simulink model "im_foc_1_1"  (R2022b)
settings: Solver=ode45  StartTime=0.0  StopTime=1  MaxStep=1e-4  MinStep=1e-5  RelTol=1e-4
values from neighbouring files (symbols this model uses):
  B = 0.00825    [IM_System_1.m]    (also in IM_System_2.m; IM_System_3.m; IM_System_noPU_4p2p2kw.m; IM_System_noPU_4p2p2kw_1.m)
  D = Ls*Lr - Lm^2    (= 0.000595276666667)    [IM_System_1.m]    (also in IM_System_2.m; IM_System_3.m; IM_System_noPU_4p2p2kw.m; IM_System_noPU_4p2p2kw_1.m)
  J = 0.013    [IM_System_1.m]    (also in IM_System_2.m; IM_System_3.m; IM_System_noPU_4p2p2kw.m; IM_System_noPU_4p2p2kw_1.m)
  Lm = 0.245/3    (= 0.0816666666667)    [IM_System_1.m]    (also in IM_System_2.m; IM_System_3.m; IM_System_noPU_4p2p2kw.m; IM_System_noPU_4p2p2kw_1.m)
  Lr = Ls    (= 0.0852333333333)    [IM_System_1.m]    (also in IM_System_2.m; IM_System_3.m; IM_System_noPU_4p2p2kw.m; IM_System_noPU_4p2p2kw_1.m)
  Ls = 0.2557/3    (= 0.0852333333333)    [IM_System_1.m]    (also in IM_System_2.m; IM_System_3.m; IM_System_noPU_4p2p2kw.m; IM_System_noPU_4p2p2kw_1.m)
  Lsigma = Ls - Lm^2/Lr    (= 0.00698408290966)    [IM_System_1.m]    (also in IM_System_2.m; IM_System_3.m; IM_System_noPU_4p2p2kw.m; IM_System_noPU_4p2p2kw_1.m)
  pole = 4    [im_params.m]
  Rr = 1.83/3    (= 0.61)    [IM_System_1.m]    (also in IM_System_2.m; IM_System_3.m; IM_System_noPU_4p2p2kw.m; IM_System_noPU_4p2p2kw_1.m)
  Rs = 2.5/3    (= 0.833333333333)    [IM_System_1.m]    (also in IM_System_2.m; IM_System_3.m; IM_System_noPU_4p2p2kw.m; IM_System_noPU_4p2p2kw_1.m)
  Tr = Lr/Rr    (= 0.139726775956)    [IM_System_1.m]    (also in IM_System_2.m; IM_System_3.m; IM_System_noPU_4p2p2kw.m; IM_System_noPU_4p2p2kw_1.m)
  w = w + iq_err*dt    (= -0.00016)    [IM_System_1.m]    (also in IM_System_2.m = -2e-05; IM_System_3.m = -2.2624e-05; IM_System_noPU_4p2p2kw.m = 0; IM_System_noPU_4p2p2kw_1.m = 0)
undefined symbols (not defined in the file or in its folder): DiscIntNeverNeededParam, sigbuilder_block, sigma
libraries: slpidlib x4
settings Model: Creator=jack  LastModifiedBy=jack

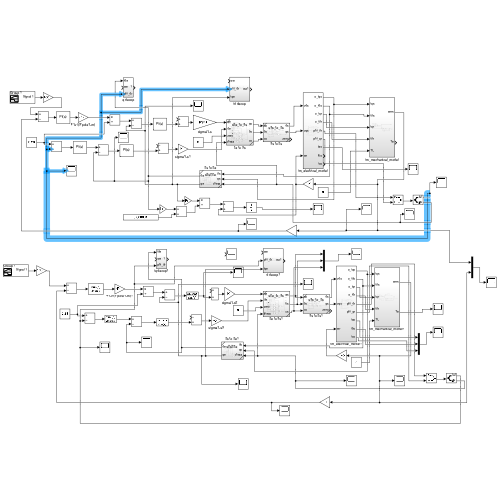
[thumbnail: Simulink's stored preview of the top-level diagram]
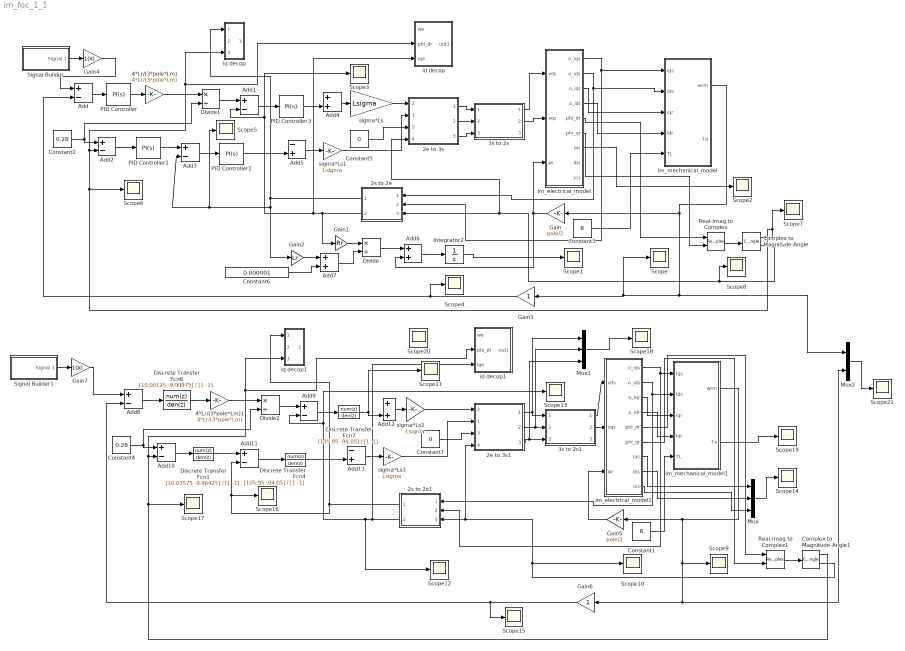
== system im_foc_1_1 ==
  2e to 3s : Subsystem  ReferencedSubsystem=s2e_to_3s
      settings: PortSchema="{\"entries\":[{\"content\":{\"sides\":[{\"content\":{\"connectorIds\":[\"In2\",\"In1\",\"In3\",\"In4\"]},\"type\":\"ConnectorPlacement.EquallySpacedRectSide\",\"uuid\":\"f133be33-91f9-49ed-9811-9ea3b8c2cc59\"},{\"content\":{\"connectorIds\":[\"Out1\",\"Out2\",\"Out3\"],\"side\":\"RIGHT\"},\"type\":\"ConnectorPlacement.EquallySpacedRectSide\",\"uuid\":\"fabe9076-6ecf-4b28-bd28-ced1febe4377\"},{\"content\":{\"connectorIds\":[],\"side\":\"TOP\"},\"type\":\"ConnectorPlacement.EquallySpacedRectSide\",\"uuid\":\"329e6c38-eee0-47c4-808c-a4969678c6ab\"}]},\"type\":\"ConnectorPlacement.EquallySpacedConnector\",\"uuid\":\"55c86aad-84a3-4804-b18d-62086c80b5dc\"}],\"packageUris\":[\"http://schema.mathworks.com/mf0/Connector/R2020b\"],\"version\":\"1.0\"}"
  2e to 3s1 : Subsystem  ReferencedSubsystem=s2e_to_3s
      settings: PortSchema="{\"entries\":[{\"content\":{\"sides\":[{\"content\":{\"connectorIds\":[\"In2\",\"In1\",\"In3\",\"In4\"]},\"type\":\"ConnectorPlacement.EquallySpacedRectSide\",\"uuid\":\"f133be33-91f9-49ed-9811-9ea3b8c2cc59\"},{\"content\":{\"connectorIds\":[\"Out1\",\"Out2\",\"Out3\"],\"side\":\"RIGHT\"},\"type\":\"ConnectorPlacement.EquallySpacedRectSide\",\"uuid\":\"fabe9076-6ecf-4b28-bd28-ced1febe4377\"},{\"content\":{\"connectorIds\":[],\"side\":\"TOP\"},\"type\":\"ConnectorPlacement.EquallySpacedRectSide\",\"uuid\":\"329e6c38-eee0-47c4-808c-a4969678c6ab\"}]},\"type\":\"ConnectorPlacement.EquallySpacedConnector\",\"uuid\":\"55c86aad-84a3-4804-b18d-62086c80b5dc\"}],\"packageUris\":[\"http://schema.mathworks.com/mf0/Connector/R2020b\"],\"version\":\"1.0\"}"
  2s to 2e : Subsystem  ReferencedSubsystem=s2s22e
  2s to 2e1 : Subsystem  ReferencedSubsystem=s2s22e
  3s to 2s : Subsystem  ReferencedSubsystem=s3s_to_2s
  3s to 2s1 : Subsystem  ReferencedSubsystem=s3s_to_2s
  4*Lr/(3*pole*Lm) : Gain  Gain=4*Lr/(3*pole*Lm)
  4*Lr/(3*pole*Lm)1 : Gain  Gain=4*Lr/(3*pole*Lm)
  Add{,1..3,8..11} (8 alike) : Sum  Inputs=+-
  Add{4,6..7,12} (4 alike) : Sum
  Add13 : Sum  Inputs=-+
  Add5 : Sum  Inputs=-+
  Complex to Magnitude-Angle : ComplexToMagnitudeAngle
  Complex to Magnitude-Angle1 : ComplexToMagnitudeAngle
  Constant1 : Constant  Value=8
  Constant2 : Constant  Value=0.28
  Constant3 : Constant  Value=8
  Constant4 : Constant  Value=0.28
  Constant5 : Constant  Value=0
  Constant6 : Constant  Value=0.000001
  Constant7 : Constant  Value=0
  Discrete Transfer Fcn1 : DiscreteTransferFcn  Numerator=[10.03575 -9.96425]  Denominator=[1 -1]  SampleTime=0.001
  Discrete Transfer Fcn4 : DiscreteTransferFcn  Numerator=[105.95 -94.05]  Denominator=[1 -1]  SampleTime=0.001
  Discrete Transfer Fcn7 : DiscreteTransferFcn  Numerator=[105.95 -94.05]  Denominator=[1 -1]  SampleTime=0.001
  Discrete Transfer Fcn8 : DiscreteTransferFcn  Numerator=[10.00125 -9.99875]  Denominator=[1 -1]  SampleTime=0.001
  Divide : Product  Inputs=*/
  Divide1 : Product  Inputs=*/
  Divide2 : Product  Inputs=*/
  Gain : Gain  Gain=pole/2
  Gain1 : Gain  Gain=Rr
  Gain2 : Gain  Gain=Lr
  Gain3 : Gain
  Gain4 : Gain  Gain=100
  Gain5 : Gain  Gain=pole/2
  Gain6 : Gain
  Gain7 : Gain  Gain=100
  Integrator2 : Integrator
  Mux : Mux  Inputs=3
  Mux1 : Mux  Inputs=3
  Mux2 : Mux  Inputs=2
  PID Controller : slpidlib/PID Controller  Controller=PI  Form=Parallel  TimeDomain=Continuous-time  UseExternalTs=off  SampleTime=-1  IntegratorMethod=Forward Euler  FilterMethod=Forward Euler  ControllerParametersSource=internal  P=10  I=0.25*10  UseKiTs=off  D=0  N=100  UseFilter=on  TunerSelectOption=Transfer Function Based (PID Tuner App)  InitialConditionSource=internal  InitialConditionForIntegrator=0  InitialConditionForFilter=0  DifferentiatorICPrevScaledInput=0  ExternalReset=none  TrackingMode=off  Kt=1  LimitOutput=off  SatLimitsSource=internal  UpperSaturationLimit=inf  LowerSaturationLimit=-inf  LinearizeAsGain=on  AntiWindupMode=none  Kb=1  LimitIntegrator=off  UpperIntegratorSaturationLimit=inf  LowerIntegratorSaturationLimit=-inf  POutMin=[]  POutMax=[]  IOutMin=[]  IOutMax=[]  DOutMin=[]  DOutMax=[]  NOutMin=[]  NOutMax=[]  SumOutMin=[]  SumOutMax=[]  SaturationOutMin=[]  SaturationOutMax=[]  PParamMin=[]  PParamMax=[]  IParamMin=[]  IParamMax=[]  DParamMin=[]  DParamMax=[]  NParamMin=[]  NParamMax=[]  KbParamMin=[]  KbParamMax=[]  KtParamMin=[]  KtParamMax=[]  KbOutMin=[]  KbOutMax=[]  KtOutMin=[]  KtOutMax=[]  IntegratorOutMin=[]  IntegratorOutMax=[]  FilterOutMin=[]  FilterOutMax=[]  SumI1OutMin=[]  SumI1OutMax=[]  SumI2OutMin=[]  SumI2OutMax=[]  SumI3OutMin=[]  SumI3OutMax=[]  SumI4OutMin=[]  SumI4OutMax=[]  SumDOutMin=[]  SumDOutMax=[]  DifferentiatorOutMin=[]  DifferentiatorOutMax=[]  FilterDiffOutCoefMin=[]  FilterDiffOutCoefMax=[]  ReciprocalOutMin=[]  ReciprocalOutMax=[]  SumDenOutMin=[]  SumDenOutMax=[]  SumNumOutMin=[]  SumNumOutMax=[]  DivideOutMin=[]  DivideOutMax=[]  UdiffTsProdOutMin=[]  UdiffTsProdOutMax=[]  NTsProdOutMin=[]  NTsProdOutMax=[]  UintegralTsProdOutMin=[]  UintegralTsProdOutMax=[]  UngainTsProdOutMin=[]  UngainTsProdOutMax=[]  ClampingZeroOutDataTypeStr=Inherit: Inherit via back propagation  ClampingZeroOutMin=[]  ClampingZeroOutMax=[]  FilterDenConstantOutDataTypeStr=Inherit: Inherit via back propagation  FilterDenConstantOutMin=[]  FilterDenConstantOutMax=[]  PCopyOutDataTypeStr=Inherit: Inherit via back propagation  PCopyOutMin=[]  PCopyOutMax=[]  NCopyOutDataTypeStr=Inherit: Inherit via back propagation  NCopyOutMin=[]  NCopyOutMax=[]  IntegratorContinuousStateAttributes=''  IntegratorStateMustResolveToSignalObject=off  IntegratorRTWStateStorageClass=Auto  FilterContinuousStateAttributes=''  FilterStateMustResolveToSignalObject=off  FilterRTWStateStorageClass=Auto  ParallelPVariant=InternalParameters  IdealPVariant=Disabled  IVariant=InternalParameters  DVariant=Disabled  IntegratorVariant=Continuous  SatVariant=Disabled  AWVariant=Passthrough  PCopyVariant=Disabled  TRVariant=Disabled  FdbkBlocksVariant=Forward  IdealPFdbkVariant=Disabled  SatFdbkVariant=Disabled  DerivativeFilterVariant=Disabled  NVariant=Disabled  NCopyVariant=Disabled_SignalSpec  FilterICVariant=Disabled  IntegratorICVariant=InternalICs  ExternalResetVariant=Disabled  TRSumVariant=Passthrough  SumFdbkVariant=Disabled  SumVariant=Sum_PI  TsampFilterVariant=InternalTs  TsampNgainVariant=Passthrough  TsampIntegralVariant=Passthrough  ExternalSaturationOutDataTypeStr=Inherit: Same as second input
  PID Controller1 : slpidlib/PID Controller  Controller=PI  Form=Parallel  TimeDomain=Continuous-time  UseExternalTs=off  SampleTime=-1  IntegratorMethod=Forward Euler  FilterMethod=Forward Euler  ControllerParametersSource=internal  P=10  I=7.15*10  UseKiTs=off  D=0  N=100  UseFilter=on  TunerSelectOption=Transfer Function Based (PID Tuner App)  InitialConditionSource=internal  InitialConditionForIntegrator=0  InitialConditionForFilter=0  DifferentiatorICPrevScaledInput=0  ExternalReset=none  TrackingMode=off  Kt=1  LimitOutput=off  SatLimitsSource=internal  UpperSaturationLimit=inf  LowerSaturationLimit=-inf  LinearizeAsGain=on  AntiWindupMode=none  Kb=1  LimitIntegrator=off  UpperIntegratorSaturationLimit=inf  LowerIntegratorSaturationLimit=-inf  POutMin=[]  POutMax=[]  IOutMin=[]  IOutMax=[]  DOutMin=[]  DOutMax=[]  NOutMin=[]  NOutMax=[]  SumOutMin=[]  SumOutMax=[]  SaturationOutMin=[]  SaturationOutMax=[]  PParamMin=[]  PParamMax=[]  IParamMin=[]  IParamMax=[]  DParamMin=[]  DParamMax=[]  NParamMin=[]  NParamMax=[]  KbParamMin=[]  KbParamMax=[]  KtParamMin=[]  KtParamMax=[]  KbOutMin=[]  KbOutMax=[]  KtOutMin=[]  KtOutMax=[]  IntegratorOutMin=[]  IntegratorOutMax=[]  FilterOutMin=[]  FilterOutMax=[]  SumI1OutMin=[]  SumI1OutMax=[]  SumI2OutMin=[]  SumI2OutMax=[]  SumI3OutMin=[]  SumI3OutMax=[]  SumI4OutMin=[]  SumI4OutMax=[]  SumDOutMin=[]  SumDOutMax=[]  DifferentiatorOutMin=[]  DifferentiatorOutMax=[]  FilterDiffOutCoefMin=[]  FilterDiffOutCoefMax=[]  ReciprocalOutMin=[]  ReciprocalOutMax=[]  SumDenOutMin=[]  SumDenOutMax=[]  SumNumOutMin=[]  SumNumOutMax=[]  DivideOutMin=[]  DivideOutMax=[]  UdiffTsProdOutMin=[]  UdiffTsProdOutMax=[]  NTsProdOutMin=[]  NTsProdOutMax=[]  UintegralTsProdOutMin=[]  UintegralTsProdOutMax=[]  UngainTsProdOutMin=[]  UngainTsProdOutMax=[]  ClampingZeroOutDataTypeStr=Inherit: Inherit via back propagation  ClampingZeroOutMin=[]  ClampingZeroOutMax=[]  FilterDenConstantOutDataTypeStr=Inherit: Inherit via back propagation  FilterDenConstantOutMin=[]  FilterDenConstantOutMax=[]  PCopyOutDataTypeStr=Inherit: Inherit via back propagation  PCopyOutMin=[]  PCopyOutMax=[]  NCopyOutDataTypeStr=Inherit: Inherit via back propagation  NCopyOutMin=[]  NCopyOutMax=[]  IntegratorContinuousStateAttributes=''  IntegratorStateMustResolveToSignalObject=off  IntegratorRTWStateStorageClass=Auto  FilterContinuousStateAttributes=''  FilterStateMustResolveToSignalObject=off  FilterRTWStateStorageClass=Auto  ParallelPVariant=InternalParameters  IdealPVariant=Disabled  IVariant=InternalParameters  DVariant=Disabled  IntegratorVariant=Continuous  SatVariant=Disabled  AWVariant=Passthrough  PCopyVariant=Disabled  TRVariant=Disabled  FdbkBlocksVariant=Forward  IdealPFdbkVariant=Disabled  SatFdbkVariant=Disabled  DerivativeFilterVariant=Disabled  NVariant=Disabled  NCopyVariant=Disabled_SignalSpec  FilterICVariant=Disabled  IntegratorICVariant=InternalICs  ExternalResetVariant=Disabled  TRSumVariant=Passthrough  SumFdbkVariant=Disabled  SumVariant=Sum_PI  TsampFilterVariant=InternalTs  TsampNgainVariant=Passthrough  TsampIntegralVariant=Passthrough  ExternalSaturationOutDataTypeStr=Inherit: Same as second input
  PID Controller2 : slpidlib/PID Controller  Controller=PI  Form=Parallel  TimeDomain=Continuous-time  UseExternalTs=off  SampleTime=-1  IntegratorMethod=Forward Euler  FilterMethod=Forward Euler  ControllerParametersSource=internal  P=100  I=119*100  UseKiTs=off  D=0  N=100  UseFilter=on  TunerSelectOption=Transfer Function Based (PID Tuner App)  InitialConditionSource=internal  InitialConditionForIntegrator=0  InitialConditionForFilter=0  DifferentiatorICPrevScaledInput=0  ExternalReset=none  TrackingMode=off  Kt=1  LimitOutput=off  SatLimitsSource=internal  UpperSaturationLimit=inf  LowerSaturationLimit=-inf  LinearizeAsGain=on  AntiWindupMode=none  Kb=1  LimitIntegrator=off  UpperIntegratorSaturationLimit=inf  LowerIntegratorSaturationLimit=-inf  POutMin=[]  POutMax=[]  IOutMin=[]  IOutMax=[]  DOutMin=[]  DOutMax=[]  NOutMin=[]  NOutMax=[]  SumOutMin=[]  SumOutMax=[]  SaturationOutMin=[]  SaturationOutMax=[]  PParamMin=[]  PParamMax=[]  IParamMin=[]  IParamMax=[]  DParamMin=[]  DParamMax=[]  NParamMin=[]  NParamMax=[]  KbParamMin=[]  KbParamMax=[]  KtParamMin=[]  KtParamMax=[]  KbOutMin=[]  KbOutMax=[]  KtOutMin=[]  KtOutMax=[]  IntegratorOutMin=[]  IntegratorOutMax=[]  FilterOutMin=[]  FilterOutMax=[]  SumI1OutMin=[]  SumI1OutMax=[]  SumI2OutMin=[]  SumI2OutMax=[]  SumI3OutMin=[]  SumI3OutMax=[]  SumI4OutMin=[]  SumI4OutMax=[]  SumDOutMin=[]  SumDOutMax=[]  DifferentiatorOutMin=[]  DifferentiatorOutMax=[]  FilterDiffOutCoefMin=[]  FilterDiffOutCoefMax=[]  ReciprocalOutMin=[]  ReciprocalOutMax=[]  SumDenOutMin=[]  SumDenOutMax=[]  SumNumOutMin=[]  SumNumOutMax=[]  DivideOutMin=[]  DivideOutMax=[]  UdiffTsProdOutMin=[]  UdiffTsProdOutMax=[]  NTsProdOutMin=[]  NTsProdOutMax=[]  UintegralTsProdOutMin=[]  UintegralTsProdOutMax=[]  UngainTsProdOutMin=[]  UngainTsProdOutMax=[]  ClampingZeroOutDataTypeStr=Inherit: Inherit via back propagation  ClampingZeroOutMin=[]  ClampingZeroOutMax=[]  FilterDenConstantOutDataTypeStr=Inherit: Inherit via back propagation  FilterDenConstantOutMin=[]  FilterDenConstantOutMax=[]  PCopyOutDataTypeStr=Inherit: Inherit via back propagation  PCopyOutMin=[]  PCopyOutMax=[]  NCopyOutDataTypeStr=Inherit: Inherit via back propagation  NCopyOutMin=[]  NCopyOutMax=[]  IntegratorContinuousStateAttributes=''  IntegratorStateMustResolveToSignalObject=off  IntegratorRTWStateStorageClass=Auto  FilterContinuousStateAttributes=''  FilterStateMustResolveToSignalObject=off  FilterRTWStateStorageClass=Auto  ParallelPVariant=InternalParameters  IdealPVariant=Disabled  IVariant=InternalParameters  DVariant=Disabled  IntegratorVariant=Continuous  SatVariant=Disabled  AWVariant=Passthrough  PCopyVariant=Disabled  TRVariant=Disabled  FdbkBlocksVariant=Forward  IdealPFdbkVariant=Disabled  SatFdbkVariant=Disabled  DerivativeFilterVariant=Disabled  NVariant=Disabled  NCopyVariant=Disabled_SignalSpec  FilterICVariant=Disabled  IntegratorICVariant=InternalICs  ExternalResetVariant=Disabled  TRSumVariant=Passthrough  SumFdbkVariant=Disabled  SumVariant=Sum_PI  TsampFilterVariant=InternalTs  TsampNgainVariant=Passthrough  TsampIntegralVariant=Passthrough  ExternalSaturationOutDataTypeStr=Inherit: Same as second input
  PID Controller3 : slpidlib/PID Controller  Controller=PI  Form=Parallel  TimeDomain=Continuous-time  UseExternalTs=off  SampleTime=-1  IntegratorMethod=Forward Euler  FilterMethod=Forward Euler  ControllerParametersSource=internal  P=100  I=119*100  UseKiTs=off  D=0  N=100  UseFilter=on  TunerSelectOption=Transfer Function Based (PID Tuner App)  InitialConditionSource=internal  InitialConditionForIntegrator=0  InitialConditionForFilter=0  DifferentiatorICPrevScaledInput=0  ExternalReset=none  TrackingMode=off  Kt=1  LimitOutput=off  SatLimitsSource=internal  UpperSaturationLimit=inf  LowerSaturationLimit=-inf  LinearizeAsGain=on  AntiWindupMode=none  Kb=1  LimitIntegrator=off  UpperIntegratorSaturationLimit=inf  LowerIntegratorSaturationLimit=-inf  POutMin=[]  POutMax=[]  IOutMin=[]  IOutMax=[]  DOutMin=[]  DOutMax=[]  NOutMin=[]  NOutMax=[]  SumOutMin=[]  SumOutMax=[]  SaturationOutMin=[]  SaturationOutMax=[]  PParamMin=[]  PParamMax=[]  IParamMin=[]  IParamMax=[]  DParamMin=[]  DParamMax=[]  NParamMin=[]  NParamMax=[]  KbParamMin=[]  KbParamMax=[]  KtParamMin=[]  KtParamMax=[]  KbOutMin=[]  KbOutMax=[]  KtOutMin=[]  KtOutMax=[]  IntegratorOutMin=[]  IntegratorOutMax=[]  FilterOutMin=[]  FilterOutMax=[]  SumI1OutMin=[]  SumI1OutMax=[]  SumI2OutMin=[]  SumI2OutMax=[]  SumI3OutMin=[]  SumI3OutMax=[]  SumI4OutMin=[]  SumI4OutMax=[]  SumDOutMin=[]  SumDOutMax=[]  DifferentiatorOutMin=[]  DifferentiatorOutMax=[]  FilterDiffOutCoefMin=[]  FilterDiffOutCoefMax=[]  ReciprocalOutMin=[]  ReciprocalOutMax=[]  SumDenOutMin=[]  SumDenOutMax=[]  SumNumOutMin=[]  SumNumOutMax=[]  DivideOutMin=[]  DivideOutMax=[]  UdiffTsProdOutMin=[]  UdiffTsProdOutMax=[]  NTsProdOutMin=[]  NTsProdOutMax=[]  UintegralTsProdOutMin=[]  UintegralTsProdOutMax=[]  UngainTsProdOutMin=[]  UngainTsProdOutMax=[]  ClampingZeroOutDataTypeStr=Inherit: Inherit via back propagation  ClampingZeroOutMin=[]  ClampingZeroOutMax=[]  FilterDenConstantOutDataTypeStr=Inherit: Inherit via back propagation  FilterDenConstantOutMin=[]  FilterDenConstantOutMax=[]  PCopyOutDataTypeStr=Inherit: Inherit via back propagation  PCopyOutMin=[]  PCopyOutMax=[]  NCopyOutDataTypeStr=Inherit: Inherit via back propagation  NCopyOutMin=[]  NCopyOutMax=[]  IntegratorContinuousStateAttributes=''  IntegratorStateMustResolveToSignalObject=off  IntegratorRTWStateStorageClass=Auto  FilterContinuousStateAttributes=''  FilterStateMustResolveToSignalObject=off  FilterRTWStateStorageClass=Auto  ParallelPVariant=InternalParameters  IdealPVariant=Disabled  IVariant=InternalParameters  DVariant=Disabled  IntegratorVariant=Continuous  SatVariant=Disabled  AWVariant=Passthrough  PCopyVariant=Disabled  TRVariant=Disabled  FdbkBlocksVariant=Forward  IdealPFdbkVariant=Disabled  SatFdbkVariant=Disabled  DerivativeFilterVariant=Disabled  NVariant=Disabled  NCopyVariant=Disabled_SignalSpec  FilterICVariant=Disabled  IntegratorICVariant=InternalICs  ExternalResetVariant=Disabled  TRSumVariant=Passthrough  SumFdbkVariant=Disabled  SumVariant=Sum_PI  TsampFilterVariant=InternalTs  TsampNgainVariant=Passthrough  TsampIntegralVariant=Passthrough  ExternalSaturationOutDataTypeStr=Inherit: Same as second input
  Real-Imag to Complex : RealImagToComplex
  Real-Imag to Complex1 : RealImagToComplex
  Scope{,1..21} (22 alike) : Scope
  Signal Builder : Subsystem  Tag=STV Subsys  LoadFcn=sigbuilder_block('load');  StartFcn=sigbuilder_block('start');  StopFcn=sigbuilder_block('stop');  ClipboardFcn=sigbuilder_block('clipboard');  mask(Sigbuilder block){tuvar=[0:10]}
      mask help: Simulink:masks:SigbuilderBlock_MD
      mask init:
      | if ~strcmp(get_param(bdroot(gcbh),'SimulationStatus'),'stopped') tuvar = sigbuilder_block('maskInit'); end
      settings: CopyFcn=sigbuilder_block('copy');  DeleteFcn=sigbuilder_block('delete');  ModelCloseFcn=sigbuilder_block('modelClose');  PreSaveFcn=sigbuilder_block('preSave');  PauseFcn=sigbuilder_block('pause');  ContinueFcn=sigbuilder_block('continue');  NameChangeFcn=sigbuilder_block('namechange');  OpenFcn=sigbuilder_block('open',[437.6 199.2 550.4 400 ]);  CloseFcn=sigbuilder_block('close');
      mask Display: plot(0, 0, 100, 100,[2, 2, 32, 32, 2], [68, 8, 8, 68, 68],[32, 2], [38, 38], [32, 19, 2],[53, 60, 44], [32, 17, 17, 2],[16, 16, 31, 31]);txt = getActiveGroup(gcbh);text(2, 100, txt,'verticalAlignment', 'top');
  Signal Builder1 : Subsystem  Tag=STV Subsys  LoadFcn=sigbuilder_block('load');  StartFcn=sigbuilder_block('start');  StopFcn=sigbuilder_block('stop');  ClipboardFcn=sigbuilder_block('clipboard');  mask(Sigbuilder block){tuvar=[0:10]}
      mask help: Simulink:masks:SigbuilderBlock_MD
      mask init:
      | if ~strcmp(get_param(bdroot(gcbh),'SimulationStatus'),'stopped') tuvar = sigbuilder_block('maskInit'); end
      settings: CopyFcn=sigbuilder_block('copy');  DeleteFcn=sigbuilder_block('delete');  ModelCloseFcn=sigbuilder_block('modelClose');  PreSaveFcn=sigbuilder_block('preSave');  PauseFcn=sigbuilder_block('pause');  ContinueFcn=sigbuilder_block('continue');  NameChangeFcn=sigbuilder_block('namechange');  OpenFcn=sigbuilder_block('open',[437.6 199.2 550.4 400 ]);  CloseFcn=sigbuilder_block('close');
      mask Display: plot(0, 0, 100, 100,[2, 2, 32, 32, 2], [68, 8, 8, 68, 68],[32, 2], [38, 38], [32, 19, 2],[53, 60, 44], [32, 17, 17, 2],[16, 16, 31, 31]);txt = getActiveGroup(gcbh);text(2, 100, txt,'verticalAlignment', 'top');
  id decop : Subsystem
  id decop1 : Subsystem
  im_electrical_model : Subsystem
  im_electrical_model1 : Subsystem
  im_mechanical_model : Subsystem
  im_mechanical_model1 : Subsystem
  iq decop : Subsystem
  iq decop1 : Subsystem
  sigma*Ls{,1..3} (4 alike) : Gain  Gain=Lsigma
  wires:
  Add/1 -> PID Controller/1
  4*Lr/(3*pole*Lm)/1 -> Divide1/1
  PID Controller/1 -> 4*Lr/(3*pole*Lm)/1
  Divide1/1 -> Add1/1
  Constant2/1 -> Add2/1, Divide1/2
  Add2/1 -> PID Controller1/1
  PID Controller1/1 -> Add3/1
  Add3/1 -> PID Controller2/1
  Add1/1 -> PID Controller3/1
  PID Controller3/1 -> Add4/2
  Add4/1 -> sigma*Ls/1
  sigma*Ls/1 -> 2e to 3s/2
  PID Controller2/1 -> Add5/2
  Add5/1 -> sigma*Ls1/1
  sigma*Ls1/1 -> 2e to 3s/1
  3s to 2s/1 -> im_electrical_model/1(vds)
  3s to 2s/2 -> im_electrical_model/2(vqs)
  im_mechanical_model/1(wrm) -> Gain/1, Scope/1, Gain3/1, Mux2/1
  im_electrical_model/1(o_iqs) -> im_mechanical_model/1(iqs), 2s to 2e/2
  im_electrical_model/2(o_ids) -> 2s to 2e/1, im_mechanical_model/2(ids)
  im_electrical_model/3(o_iqr) -> im_mechanical_model/3(iqr)
  im_electrical_model/4(o_idr) -> im_mechanical_model/4(idr)
  2s to 2e/1 -> iq decop/1(ide), Gain2/1, Scope5/1, Add3/2
  2s to 2e/2 -> id decop/3(iqe), Scope3/1, Add1/2, Gain1/1
  Gain1/1 -> Divide/1
  Divide/1 -> Add6/1
  Gain/1 -> im_electrical_model/3(wr), Add6/2
  Add6/1 -> Integrator2/1
  Integrator2/1 -> Scope1/1
  Constant5/1 -> 2e to 3s/3
  Gain2/1 -> Add7/1
  Add7/1 -> Divide/2
  Constant6/1 -> Add7/2
  2e to 3s/1 -> 3s to 2s/1
  2e to 3s/3 -> 3s to 2s/3
  im_electrical_model/7(ias) -> Scope2/1
  Gain3/1 -> Scope4/1, Add/2
  2e to 3s/2 -> 3s to 2s/2
  Signal Builder/1(Signal 1) -> Gain4/1
  Complex to Magnitude-Angle/1 -> Scope6/1, id decop/2(phi_dr), iq decop/3(phi_dr), Add2/2, Scope7/1
  Constant3/1 -> im_mechanical_model/5(TL)
  Gain4/1 -> Add/1
  im_electrical_model/5(phi_dr) -> Real-Imag to Complex/1
  im_electrical_model/6(phi_qr) -> Real-Imag to Complex/2
  Real-Imag to Complex/1 -> Complex to Magnitude-Angle/1
  Complex to Magnitude-Angle/2 -> Scope8/1, 2e to 3s/4, 2s to 2e/3
  Real-Imag to Complex1/1 -> Complex to Magnitude-Angle1/1
  3s to 2s1/2 -> im_electrical_model1/2(vqs)
  Signal Builder1/1(Signal 1) -> Gain7/1
  Constant4/1 -> Add10/1, Divide2/2
  im_electrical_model1/3(o_iqr) -> im_mechanical_model1/3(iqr)
  Discrete Transfer Fcn1/1 -> Add11/1
  im_electrical_model1/1(o_iqs) -> im_mechanical_model1/1(iqs), 2s to 2e1/2
  im_electrical_model1/5(phi_dr) -> Real-Imag to Complex1/1
  2s to 2e1/2 -> Scope12/1, Scope13/1, Add9/2, id decop1/3(iqe)
  Add9/1 -> Discrete Transfer Fcn7/1
  im_mechanical_model1/1(wrm) -> Gain5/1, Gain6/1, Mux2/2, Scope9/1
  2s to 2e1/1 -> iq decop1/1(ide), Scope16/1, Add11/2
  im_electrical_model1/2(o_ids) -> 2s to 2e1/1, im_mechanical_model1/2(ids)
  Discrete Transfer Fcn4/1 -> Add13/2
  Add12/1 -> sigma*Ls2/1
  2e to 3s1/1 -> Mux1/1, 3s to 2s1/1
  Add8/1 -> Discrete Transfer Fcn8/1
  4*Lr/(3*pole*Lm)1/1 -> Divide2/1
  Constant1/1 -> im_mechanical_model1/5(TL)
  Add13/1 -> sigma*Ls3/1
  im_electrical_model1/4(o_idr) -> im_mechanical_model1/4(idr)
  Discrete Transfer Fcn7/1 -> Scope11/1, Add12/2
  Gain5/1 -> im_electrical_model1/3(wr)
  sigma*Ls2/1 -> 2e to 3s1/2
  Constant7/1 -> 2e to 3s1/3
  Add10/1 -> Discrete Transfer Fcn1/1
  Complex to Magnitude-Angle1/2 -> 2e to 3s1/4, 2s to 2e1/3, Scope10/1
  im_electrical_model1/9(ics) -> Mux/3
  Add11/1 -> Discrete Transfer Fcn4/1
  2e to 3s1/3 -> Mux1/3, 3s to 2s1/3
  im_electrical_model1/7(ias) -> Mux/1
  im_electrical_model1/6(phi_qr) -> Real-Imag to Complex1/2
  im_electrical_model1/8(ibs) -> Mux/2
  Mux/1 -> Scope14/1
  Discrete Transfer Fcn8/1 -> 4*Lr/(3*pole*Lm)1/1
  Mux1/1 -> Scope18/1
  Gain6/1 -> Scope15/1, Add8/2
  3s to 2s1/1 -> im_electrical_model1/1(vds)
  Gain7/1 -> Add8/1
  2e to 3s1/2 -> Mux1/2, 3s to 2s1/2
  im_mechanical_model1/2(Te) -> Scope19/1
  Divide2/1 -> Add9/1
  Complex to Magnitude-Angle1/1 -> Scope17/1, id decop1/2(phi_dr), iq decop1/3(phi_dr), Add10/2
  sigma*Ls3/1 -> 2e to 3s1/1
  Mux2/1 -> Scope21/1

== system im_foc_1_1/Signal Builder ==
  Demux : Demux  Tag=STV Demux  Outputs=1
      settings: DisplayOption=none
  FromWs : FromWorkspace  Tag=STV FromWs  VariableName=tuvar
      SigBuilderData=|
      | common.afterFinalStr = 'Extrapolate'
      | common.sampleTime = 0
      | dataSet.timeRange = [0 10]
      | dataSet.name = 'Group 1'
      | sbobj.Groups.Name = 'Group 1'
      | sbobj.Groups.Signals.Name = 'Signal 1'
      | sbobj.Groups.Signals.XData = [0 0.5 4 6 6 10]
      | sbobj.Groups.Signals.YData = [0 1 1 1 0 0]
  Signal 1 : Outport  Tag=STV Outport
  wires:
  Demux/1 -> Signal 1/1
  FromWs/1 -> Demux/1

== system im_foc_1_1/Signal Builder1 ==
  Demux : Demux  Tag=STV Demux  Outputs=1
      settings: DisplayOption=none
  FromWs : FromWorkspace  Tag=STV FromWs  VariableName=tuvar
      SigBuilderData=|
      | common.afterFinalStr = 'Extrapolate'
      | common.sampleTime = 0
      | dataSet.timeRange = [0 10]
      | dataSet.name = 'Group 1'
      | sbobj.Groups.Name = 'Group 1'
      | sbobj.Groups.Signals.Name = 'Signal 1'
      | sbobj.Groups.Signals.XData = [0 0.5 4 6 6 10]
      | sbobj.Groups.Signals.YData = [0 1 1 1 0 0]
  Signal 1 : Outport  Tag=STV Outport
  wires:
  Demux/1 -> Signal 1/1
  FromWs/1 -> Demux/1

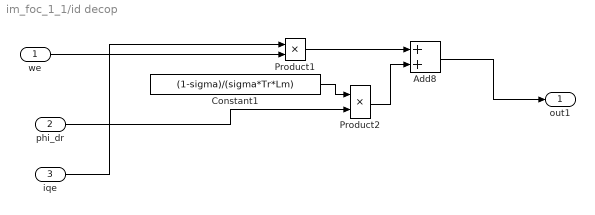
== system im_foc_1_1/id decop ==
  we : Inport
  phi_dr : Inport  Port=2
  iqe : Inport  Port=3
  Add8 : Sum
  Constant1 : Constant  Value=(1-sigma)/(sigma*Tr*Lm)
  Product1 : Product
  Product2 : Product
  out1 : Outport
  wires:
  Product1/1 -> Add8/1
  iqe/1 -> Product1/1
  Add8/1 -> out1/1
  we/1 -> Product1/2
  Constant1/1 -> Product2/1
  Product2/1 -> Add8/2
  phi_dr/1 -> Product2/2

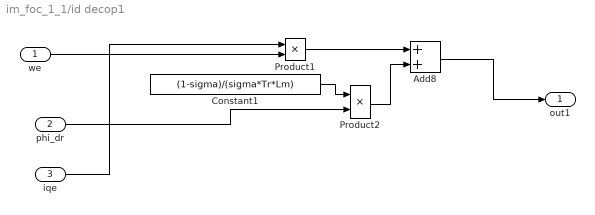
== system im_foc_1_1/id decop1 ==
  we : Inport
  phi_dr : Inport  Port=2
  iqe : Inport  Port=3
  Add8 : Sum
  Constant1 : Constant  Value=(1-sigma)/(sigma*Tr*Lm)
  Product1 : Product
  Product2 : Product
  out1 : Outport
  wires:
  Product1/1 -> Add8/1
  iqe/1 -> Product1/1
  Add8/1 -> out1/1
  we/1 -> Product1/2
  Constant1/1 -> Product2/1
  Product2/1 -> Add8/2
  phi_dr/1 -> Product2/2

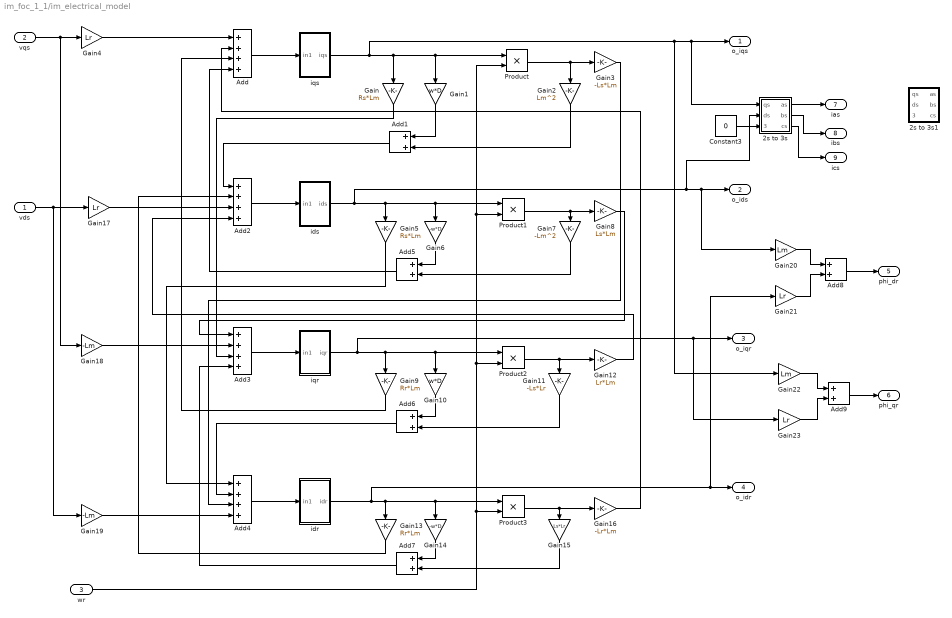
== system im_foc_1_1/im_electrical_model ==
  vds : Inport
  vqs : Inport  Port=2
  wr : Inport  Port=3
  2s to 3s : Subsystem
  2s to 3s1 : Subsystem
  Add{,2..4} (4 alike) : Sum  Inputs=++++
  Add{1,5..9} (6 alike) : Sum
  Constant3 : Constant  Value=0
  Gain : Gain  Gain=Rs*Lm
  Gain1 : Gain  Gain=w*D
  Gain10 : Gain  Gain=w*D
  Gain11 : Gain  Gain=-Ls*Lr
  Gain12 : Gain  Gain=Lr*Lm
  Gain13 : Gain  Gain=Rr*Lm
  Gain14 : Gain  Gain=-w*D
  Gain15 : Gain  Gain=Ls*Lr
  Gain16 : Gain  Gain=-Lr*Lm
  Gain{4,17,21,23} (4 alike) : Gain  Gain=Lr
  Gain18 : Gain  Gain=-Lm
  Gain19 : Gain  Gain=-Lm
  Gain2 : Gain  Gain=Lm^2
  Gain20 : Gain  Gain=Lm
  Gain22 : Gain  Gain=Lm
  Gain3 : Gain  Gain=-Ls*Lm
  Gain5 : Gain  Gain=Rs*Lm
  Gain6 : Gain  Gain=-w*D
  Gain7 : Gain  Gain=-Lm^2
  Gain8 : Gain  Gain=Ls*Lm
  Gain9 : Gain  Gain=Rr*Lm
  Product{,1..3} (4 alike) : Product
  idr : Subsystem
  ids : Subsystem
  iqr : Subsystem
  iqs : Subsystem
  o_iqs : Outport
  o_ids : Outport  Port=2
  o_iqr : Outport  Port=3
  o_idr : Outport  Port=4
  phi_dr : Outport  Port=5
  phi_qr : Outport  Port=6
  ias : Outport  Port=7
  ibs : Outport  Port=8
  ics : Outport  Port=9
  wires:
  Add/1 -> iqs/1(in1)
  iqs/1(iqs) -> Gain22/1, 2s to 3s/1(qs), o_iqs/1, Gain1/1, Product/1, Gain/1
  Gain1/1 -> Add1/1
  Product/1 -> Gain3/1, Gain2/1
  Gain2/1 -> Add1/2
  Gain/1 -> Add3/3
  Add1/1 -> Add2/1
  Gain4/1 -> Add/1
  vqs/1 -> Gain18/1, Gain4/1
  wr/1 -> Product3/2, Product2/2, Product1/2, Product/2
  Add2/1 -> ids/1(in1)
  Product1/1 -> Gain7/1, Gain8/1
  ids/1(ids) -> 2s to 3s/2(ds), Gain20/1, o_ids/1, Gain5/1, Gain6/1, Product1/1
  Gain5/1 -> Add4/1
  Gain6/1 -> Add5/1
  Gain7/1 -> Add5/2
  Add5/1 -> Add/4
  Gain8/1 -> Add3/1
  iqr/1(iqr) -> Gain23/1, o_iqr/1, Gain9/1, Gain10/1, Product2/1
  Product2/1 -> Gain11/1, Gain12/1
  Gain10/1 -> Add6/1
  Gain11/1 -> Add6/2
  Add6/1 -> Add4/2
  Gain9/1 -> Add/3
  Gain12/1 -> Add2/4
  Add3/1 -> iqr/1(in1)
  idr/1(idr) -> Gain21/1, o_idr/1, Product3/1, Gain14/1, Gain13/1
  Gain14/1 -> Add7/1
  Gain15/1 -> Add7/2
  Product3/1 -> Gain15/1, Gain16/1
  Gain16/1 -> Add/2
  Add7/1 -> Add3/4
  Add4/1 -> idr/1(in1)
  Gain13/1 -> Add2/2
  Gain3/1 -> Add4/3
  vds/1 -> Gain19/1, Gain17/1
  Gain19/1 -> Add4/4
  Gain18/1 -> Add3/2
  Gain17/1 -> Add2/3
  Gain20/1 -> Add8/1
  Gain21/1 -> Add8/2
  Add8/1 -> phi_dr/1
  Gain23/1 -> Add9/2
  Gain22/1 -> Add9/1
  Add9/1 -> phi_qr/1
  Constant3/1 -> 2s to 3s/3(zero)
  2s to 3s/1(as) -> ias/1
  2s to 3s/2(bs) -> ibs/1
  2s to 3s/3(cs) -> ics/1

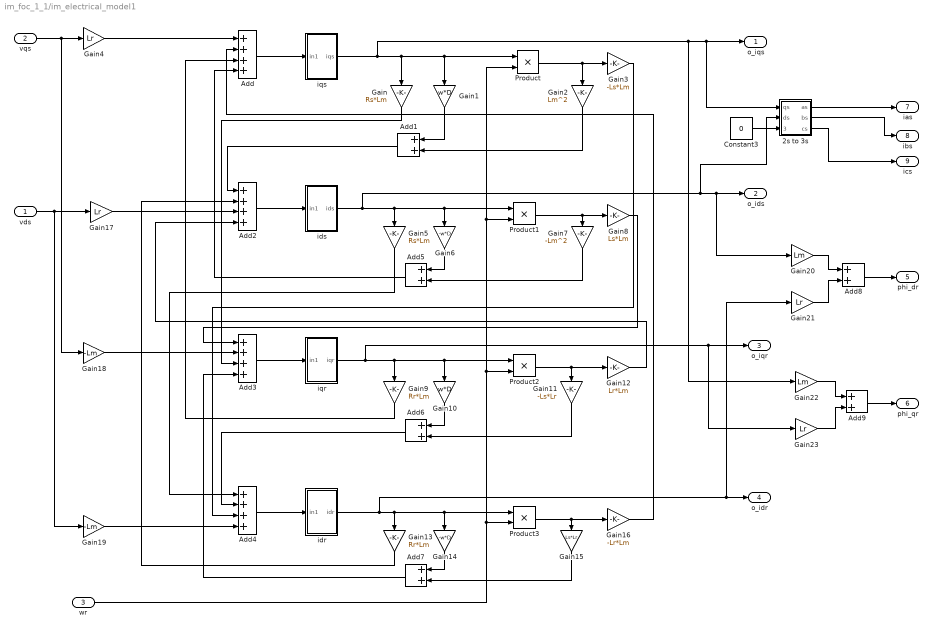
== system im_foc_1_1/im_electrical_model1 ==
  vds : Inport
  vqs : Inport  Port=2
  wr : Inport  Port=3
  2s to 3s : Subsystem
  Add{,2..4} (4 alike) : Sum  Inputs=++++
  Add{1,5..9} (6 alike) : Sum
  Constant3 : Constant  Value=0
  Gain : Gain  Gain=Rs*Lm
  Gain1 : Gain  Gain=w*D
  Gain10 : Gain  Gain=w*D
  Gain11 : Gain  Gain=-Ls*Lr
  Gain12 : Gain  Gain=Lr*Lm
  Gain13 : Gain  Gain=Rr*Lm
  Gain14 : Gain  Gain=-w*D
  Gain15 : Gain  Gain=Ls*Lr
  Gain16 : Gain  Gain=-Lr*Lm
  Gain{4,17,21,23} (4 alike) : Gain  Gain=Lr
  Gain18 : Gain  Gain=-Lm
  Gain19 : Gain  Gain=-Lm
  Gain2 : Gain  Gain=Lm^2
  Gain20 : Gain  Gain=Lm
  Gain22 : Gain  Gain=Lm
  Gain3 : Gain  Gain=-Ls*Lm
  Gain5 : Gain  Gain=Rs*Lm
  Gain6 : Gain  Gain=-w*D
  Gain7 : Gain  Gain=-Lm^2
  Gain8 : Gain  Gain=Ls*Lm
  Gain9 : Gain  Gain=Rr*Lm
  Product{,1..3} (4 alike) : Product
  idr : Subsystem
  ids : Subsystem
  iqr : Subsystem
  iqs : Subsystem
  o_iqs : Outport
  o_ids : Outport  Port=2
  o_iqr : Outport  Port=3
  o_idr : Outport  Port=4
  phi_dr : Outport  Port=5
  phi_qr : Outport  Port=6
  ias : Outport  Port=7
  ibs : Outport  Port=8
  ics : Outport  Port=9
  wires:
  Add/1 -> iqs/1(in1)
  iqs/1(iqs) -> Gain22/1, 2s to 3s/1(qs), o_iqs/1, Gain1/1, Product/1, Gain/1
  Gain1/1 -> Add1/1
  Product/1 -> Gain3/1, Gain2/1
  Gain2/1 -> Add1/2
  Gain/1 -> Add3/3
  Add1/1 -> Add2/1
  Gain4/1 -> Add/1
  vqs/1 -> Gain18/1, Gain4/1
  wr/1 -> Product3/2, Product2/2, Product1/2, Product/2
  Add2/1 -> ids/1(in1)
  Product1/1 -> Gain7/1, Gain8/1
  ids/1(ids) -> 2s to 3s/2(ds), Gain20/1, o_ids/1, Gain5/1, Gain6/1, Product1/1
  Gain5/1 -> Add4/1
  Gain6/1 -> Add5/1
  Gain7/1 -> Add5/2
  Add5/1 -> Add/4
  Gain8/1 -> Add3/1
  iqr/1(iqr) -> Gain23/1, o_iqr/1, Gain9/1, Gain10/1, Product2/1
  Product2/1 -> Gain11/1, Gain12/1
  Gain10/1 -> Add6/1
  Gain11/1 -> Add6/2
  Add6/1 -> Add4/2
  Gain9/1 -> Add/3
  Gain12/1 -> Add2/4
  Add3/1 -> iqr/1(in1)
  idr/1(idr) -> Gain21/1, o_idr/1, Product3/1, Gain14/1, Gain13/1
  Gain14/1 -> Add7/1
  Gain15/1 -> Add7/2
  Product3/1 -> Gain15/1, Gain16/1
  Gain16/1 -> Add/2
  Add7/1 -> Add3/4
  Add4/1 -> idr/1(in1)
  Gain13/1 -> Add2/2
  Gain3/1 -> Add4/3
  vds/1 -> Gain19/1, Gain17/1
  Gain19/1 -> Add4/4
  Gain18/1 -> Add3/2
  Gain17/1 -> Add2/3
  Gain20/1 -> Add8/1
  Gain21/1 -> Add8/2
  Add8/1 -> phi_dr/1
  Gain23/1 -> Add9/2
  Gain22/1 -> Add9/1
  Add9/1 -> phi_qr/1
  Constant3/1 -> 2s to 3s/3(zero)
  2s to 3s/1(as) -> ias/1
  2s to 3s/2(bs) -> ibs/1
  2s to 3s/3(cs) -> ics/1

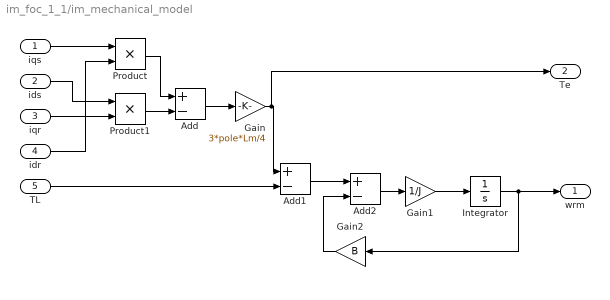
== system im_foc_1_1/im_mechanical_model ==
  iqs : Inport
  ids : Inport  Port=2
  iqr : Inport  Port=3
  idr : Inport  Port=4
  TL : Inport  Port=5
  Add : Sum  Inputs=+-
  Add1 : Sum  Inputs=+-
  Add2 : Sum  Inputs=+-
  Gain : Gain  Gain=3*pole*Lm/4
  Gain1 : Gain  Gain=1/J
  Gain2 : Gain  Gain=B
  Integrator : Integrator
  Product : Product
  Product1 : Product
  wrm : Outport
  Te : Outport  Port=2
  wires:
  Add1/1 -> Add2/1
  iqr/1 -> Product1/2
  idr/1 -> Product/2
  TL/1 -> Add1/2
  iqs/1 -> Product/1
  Product/1 -> Add/1
  Add/1 -> Gain/1
  ids/1 -> Product1/1
  Add2/1 -> Gain1/1
  Gain1/1 -> Integrator/1
  Product1/1 -> Add/2
  Gain2/1 -> Add2/2
  Gain/1 -> Te/1, Add1/1
  Integrator/1 -> wrm/1, Gain2/1

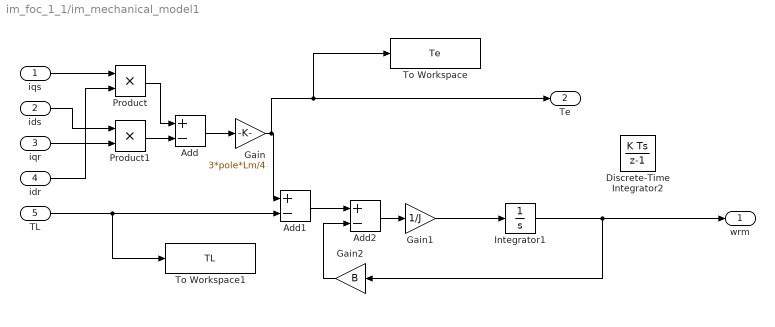
== system im_foc_1_1/im_mechanical_model1 ==
  iqs : Inport
  ids : Inport  Port=2
  iqr : Inport  Port=3
  idr : Inport  Port=4
  TL : Inport  Port=5
  Add : Sum  Inputs=+-
  Add1 : Sum  Inputs=+-
  Add2 : Sum  Inputs=+-
  Discrete-Time Integrator2 : DiscreteIntegrator  SampleTime=-1  ICPrevOutput=DiscIntNeverNeededParam  ICPrevScaledInput=DiscIntNeverNeededParam
  Gain : Gain  Gain=3*pole*Lm/4
  Gain1 : Gain  Gain=1/J
  Gain2 : Gain  Gain=B
  Integrator1 : Integrator
  Product : Product
  Product1 : Product
  To Workspace : ToWorkspace  VariableName=Te  SaveFormat=Timeseries  SampleTime=-1
  To Workspace1 : ToWorkspace  VariableName=TL  SaveFormat=Timeseries  SampleTime=-1
  wrm : Outport
  Te : Outport  Port=2
  wires:
  Add1/1 -> Add2/1
  iqr/1 -> Product1/2
  idr/1 -> Product/2
  TL/1 -> To Workspace1/1, Add1/2
  iqs/1 -> Product/1
  Product/1 -> Add/1
  Add/1 -> Gain/1
  ids/1 -> Product1/1
  Add2/1 -> Gain1/1
  Product1/1 -> Add/2
  Gain2/1 -> Add2/2
  Gain/1 -> To Workspace/1, Te/1, Add1/1
  Gain1/1 -> Integrator1/1
  Integrator1/1 -> Gain2/1, wrm/1

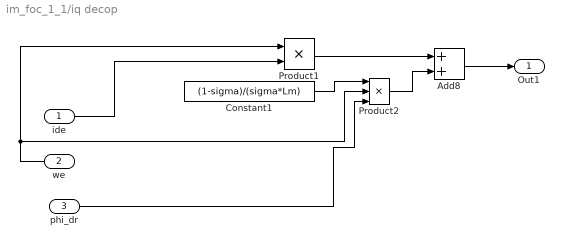
== system im_foc_1_1/iq decop ==
  ide : Inport
  we : Inport  Port=2
  phi_dr : Inport  Port=3
  Add8 : Sum
  Constant1 : Constant  Value=(1-sigma)/(sigma*Lm)
  Product1 : Product
  Product2 : Product  Inputs=3
  Out1 : Outport
  wires:
  Add8/1 -> Out1/1
  phi_dr/1 -> Product2/3
  we/1 -> Product2/2, Product1/1
  Constant1/1 -> Product2/1
  Product2/1 -> Add8/2
  ide/1 -> Product1/2
  Product1/1 -> Add8/1

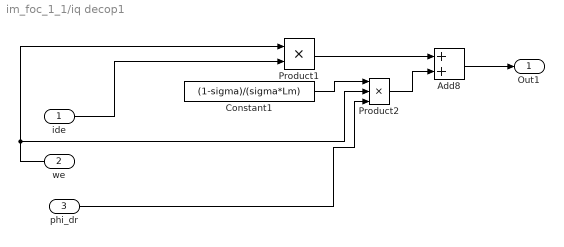
== system im_foc_1_1/iq decop1 ==
  ide : Inport
  we : Inport  Port=2
  phi_dr : Inport  Port=3
  Add8 : Sum
  Constant1 : Constant  Value=(1-sigma)/(sigma*Lm)
  Product1 : Product
  Product2 : Product  Inputs=3
  Out1 : Outport
  wires:
  Add8/1 -> Out1/1
  phi_dr/1 -> Product2/3
  we/1 -> Product2/2, Product1/1
  Constant1/1 -> Product2/1
  Product2/1 -> Add8/2
  ide/1 -> Product1/2
  Product1/1 -> Add8/1

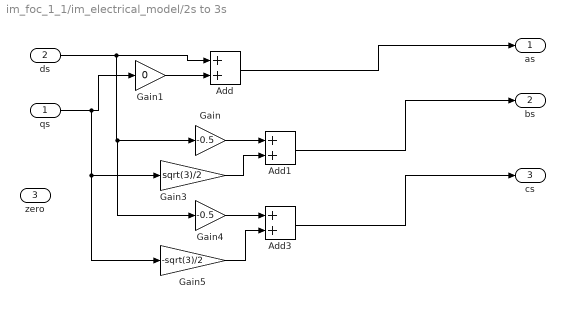
== system im_foc_1_1/im_electrical_model/2s to 3s ==
  qs : Inport
  ds : Inport  Port=2
  zero : Inport  Port=3
  Add : Sum
  Add1 : Sum
  Add3 : Sum
  Gain : Gain  Gain=-0.5
  Gain1 : Gain  Gain=0
  Gain3 : Gain  Gain=sqrt(3)/2
  Gain4 : Gain  Gain=-0.5
  Gain5 : Gain  Gain=-sqrt(3)/2
  as : Outport
  bs : Outport  Port=2
  cs : Outport  Port=3
  wires:
  ds/1 -> Gain4/1, Gain/1, Add/1
  qs/1 -> Gain5/1, Gain3/1, Gain1/1
  Gain1/1 -> Add/2
  Gain/1 -> Add1/1
  Gain3/1 -> Add1/2
  Gain4/1 -> Add3/1
  Gain5/1 -> Add3/2
  Add/1 -> as/1
  Add1/1 -> bs/1
  Add3/1 -> cs/1

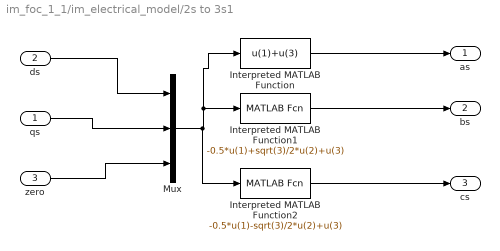
== system im_foc_1_1/im_electrical_model/2s to 3s1 ==
  qs : Inport
  ds : Inport  Port=2
  zero : Inport  Port=3
  Interpreted MATLAB Function : MATLABFcn  MATLABFcn=u(1)+u(3)
  Interpreted MATLAB Function1 : MATLABFcn  MATLABFcn=-0.5*u(1)+sqrt(3)/2*u(2)+u(3)
  Interpreted MATLAB Function2 : MATLABFcn  MATLABFcn=-0.5*u(1)-sqrt(3)/2*u(2)+u(3)
  Mux : Mux  Inputs=3
  as : Outport
  bs : Outport  Port=2
  cs : Outport  Port=3
  wires:
  Interpreted MATLAB Function1/1 -> bs/1
  Interpreted MATLAB Function/1 -> as/1
  Interpreted MATLAB Function2/1 -> cs/1
  zero/1 -> Mux/3
  Mux/1 -> Interpreted MATLAB Function2/1, Interpreted MATLAB Function/1, Interpreted MATLAB Function1/1
  ds/1 -> Mux/1
  qs/1 -> Mux/2

== system im_foc_1_1/im_electrical_model/idr ==
  in1 : Inport
  Add : Sum  Inputs=+-
  Gain : Gain  Gain=1/D
  Gain1 : Gain  Gain=Rr*Ls
  Integrator : Integrator
  idr : Outport
  wires:
  in1/1 -> Add/1
  Gain1/1 -> Add/2
  Gain/1 -> Integrator/1
  Integrator/1 -> idr/1, Gain1/1
  Add/1 -> Gain/1

== system im_foc_1_1/im_electrical_model/ids ==
  in1 : Inport
  Add : Sum  Inputs=+-
  Gain : Gain  Gain=1/D
  Gain1 : Gain  Gain=Rs*Lr
  Integrator : Integrator
  ids : Outport
  wires:
  Gain1/1 -> Add/2
  Gain/1 -> Integrator/1
  Add/1 -> Gain/1
  in1/1 -> Add/1
  Integrator/1 -> ids/1, Gain1/1

== system im_foc_1_1/im_electrical_model/iqr ==
  in1 : Inport
  Add : Sum  Inputs=+-
  Gain : Gain  Gain=1/D
  Gain1 : Gain  Gain=Rr*Ls
  Integrator : Integrator
  iqr : Outport
  wires:
  in1/1 -> Add/1
  Gain/1 -> Integrator/1
  Gain1/1 -> Add/2
  Add/1 -> Gain/1
  Integrator/1 -> iqr/1, Gain1/1

== system im_foc_1_1/im_electrical_model/iqs ==
  in1 : Inport
  Add : Sum  Inputs=+-
  Gain : Gain  Gain=1/D
  Gain1 : Gain  Gain=Rs*Lr
  Integrator : Integrator
  iqs : Outport
  wires:
  Gain/1 -> Integrator/1
  Add/1 -> Gain/1
  in1/1 -> Add/1
  Gain1/1 -> Add/2
  Integrator/1 -> iqs/1, Gain1/1

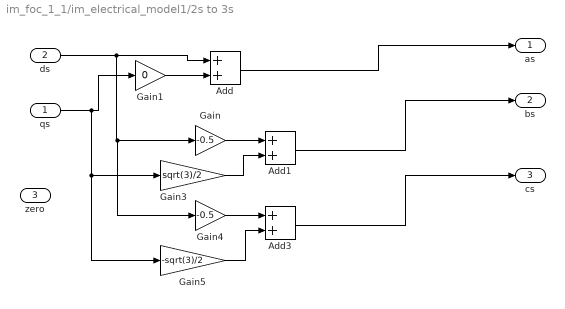
== system im_foc_1_1/im_electrical_model1/2s to 3s ==
  qs : Inport
  ds : Inport  Port=2
  zero : Inport  Port=3
  Add : Sum
  Add1 : Sum
  Add3 : Sum
  Gain : Gain  Gain=-0.5
  Gain1 : Gain  Gain=0
  Gain3 : Gain  Gain=sqrt(3)/2
  Gain4 : Gain  Gain=-0.5
  Gain5 : Gain  Gain=-sqrt(3)/2
  as : Outport
  bs : Outport  Port=2
  cs : Outport  Port=3
  wires:
  ds/1 -> Gain4/1, Gain/1, Add/1
  qs/1 -> Gain5/1, Gain3/1, Gain1/1
  Gain1/1 -> Add/2
  Gain/1 -> Add1/1
  Gain3/1 -> Add1/2
  Gain4/1 -> Add3/1
  Gain5/1 -> Add3/2
  Add/1 -> as/1
  Add1/1 -> bs/1
  Add3/1 -> cs/1

== system im_foc_1_1/im_electrical_model1/idr ==
  in1 : Inport
  Add : Sum  Inputs=+-
  Discrete-Time Integrator1 : DiscreteIntegrator  SampleTime=-1  ICPrevOutput=DiscIntNeverNeededParam  ICPrevScaledInput=DiscIntNeverNeededParam
  Gain : Gain  Gain=1/D
  Gain1 : Gain  Gain=Rr*Ls
  Integrator2 : Integrator
  idr : Outport
  wires:
  in1/1 -> Add/1
  Gain1/1 -> Add/2
  Gain/1 -> Integrator2/1
  Integrator2/1 -> idr/1, Gain1/1
  Add/1 -> Gain/1

== system im_foc_1_1/im_electrical_model1/ids ==
  in1 : Inport
  Add : Sum  Inputs=+-
  Discrete-Time Integrator2 : DiscreteIntegrator  SampleTime=-1  ICPrevOutput=DiscIntNeverNeededParam  ICPrevScaledInput=DiscIntNeverNeededParam
  Gain : Gain  Gain=1/D
  Gain1 : Gain  Gain=Rs*Lr
  Integrator2 : Integrator
  ids : Outport
  wires:
  Gain1/1 -> Add/2
  Gain/1 -> Integrator2/1
  Add/1 -> Gain/1
  in1/1 -> Add/1
  Integrator2/1 -> ids/1, Gain1/1

== system im_foc_1_1/im_electrical_model1/iqr ==
  in1 : Inport
  Add : Sum  Inputs=+-
  Discrete-Time Integrator2 : DiscreteIntegrator  SampleTime=-1  ICPrevOutput=DiscIntNeverNeededParam  ICPrevScaledInput=DiscIntNeverNeededParam
  Gain : Gain  Gain=1/D
  Gain1 : Gain  Gain=Rr*Ls
  Integrator2 : Integrator
  iqr : Outport
  wires:
  in1/1 -> Add/1
  Gain/1 -> Integrator2/1
  Gain1/1 -> Add/2
  Add/1 -> Gain/1
  Integrator2/1 -> iqr/1, Gain1/1

== system im_foc_1_1/im_electrical_model1/iqs ==
  in1 : Inport
  Add : Sum  Inputs=+-
  Discrete-Time Integrator1 : DiscreteIntegrator  SampleTime=-1  ICPrevOutput=DiscIntNeverNeededParam  ICPrevScaledInput=DiscIntNeverNeededParam
  Gain : Gain  Gain=1/D
  Gain1 : Gain  Gain=Rs*Lr
  Integrator2 : Integrator
  iqs : Outport
  wires:
  Add/1 -> Gain/1
  in1/1 -> Add/1
  Gain1/1 -> Add/2
  Gain/1 -> Integrator2/1
  Integrator2/1 -> Gain1/1, iqs/1
